simulink model "motor"  (R2017b)
settings: Solver=VariableStepAuto  StartTime=0.0  StopTime=12  FixedStep=0.001  RelTol=1e-3
undefined symbols (not defined in the file or in its folder): Amp1d, Amp1n, AmpSat1, BackEMF1, DiscIntNeverNeededParam, Elec1d, Elec1n, Mech1d, Mech1n, NomCurrent, PWMConversion, StallCurrent, StaticFric, TConst1
libraries: simulink x10
settings Model: SimulationMode=accelerator  Creator=Moochster  LastModifiedBy=lucyl

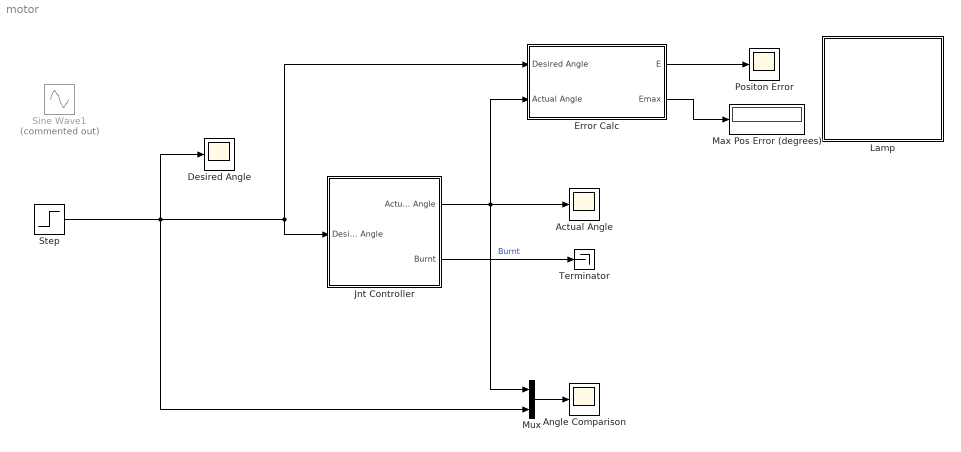
== system motor ==
  Actual Angle : Scope
  Angle Comparison : Scope
  Desired Angle : Scope
  Error Calc : Subsystem
  Jnt Controller : Subsystem
  Lamp : Subsystem  DialogController=hmiCreateDDGDialog  IsWebBlock=on  mask(MWDashboardBlock){webBlockId=7fcfd6b5-b98b-441a-9880-35fe4990fbef, webBlockType=lamp, ShowInLibBrowser=on, ShowInitialText=on, HMISrcModelName=motor}
      mask prompts: webBlockType "WebBlock Type"; HMISrcModelName "Source Model"
      mask help: SimulinkHMI:dialogs:LampDialogDesc
      mask Help: helpview([docroot '/mapfiles/simulink.map'], 'hmi_lamp')
      mask Display:
      | if strcmp(get_param(bdroot(gcb),'BlockDiagramType'), 'library')
      |     image([(matlabroot) '/toolbox/simulink/hmi/icons/Lamp.png']);
      | end
  Max Pos Error (degrees) : Display
  Mux : Mux  Inputs=2
  Positon Error : Scope
  Sine Wave1 : Sin  Commented=on  Amplitude=pi/4  Frequency=15*2*pi  Samples=15  SampleTime=0
  Step : Step  Time=0.02  SampleTime=0
  Terminator : Terminator
  wires:
  Step/1 -> Mux/2, Desired Angle/1, Error Calc/1(Desired Angle), Jnt Controller/1(Desired Angle)
  Jnt Controller/1(Actual Angle) -> Error Calc/2(Actual Angle), Actual Angle/1, Mux/1
  Error Calc/1(E) -> Positon Error/1
  Error Calc/2(Emax) -> Max Pos Error (degrees)/1
  Jnt Controller/2(Burnt) -> Terminator/1  "Burnt"
  Mux/1 -> Angle Comparison/1

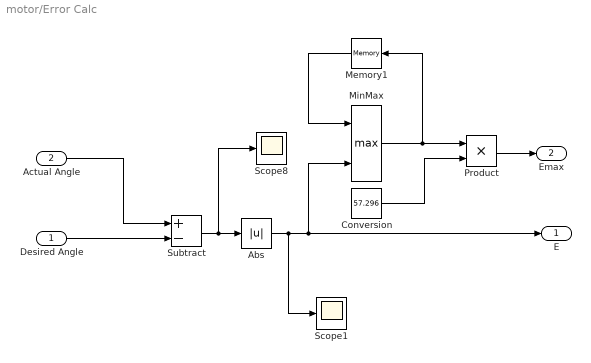
== system motor/Error Calc ==
  Desired Angle : Inport
  Actual Angle : Inport  Port=2
  Abs : Abs
  Conversion : Constant  Value=57.296
  Memory1 : Memory
  MinMax : MinMax  Function=max  Inputs=2  ZeroCross=off
  Product : Product
  Scope1 : Scope
  Scope8 : Scope
  Subtract : Sum  Inputs=+-
  E : Outport
  Emax : Outport  Port=2
  wires:
  Actual Angle/1 -> Subtract/1
  Desired Angle/1 -> Subtract/2
  Subtract/1 -> Scope8/1, Abs/1
  MinMax/1 -> Product/1, Memory1/1
  Memory1/1 -> MinMax/1
  Abs/1 -> Scope1/1, MinMax/2, E/1
  Product/1 -> Emax/1
  Conversion/1 -> Product/2

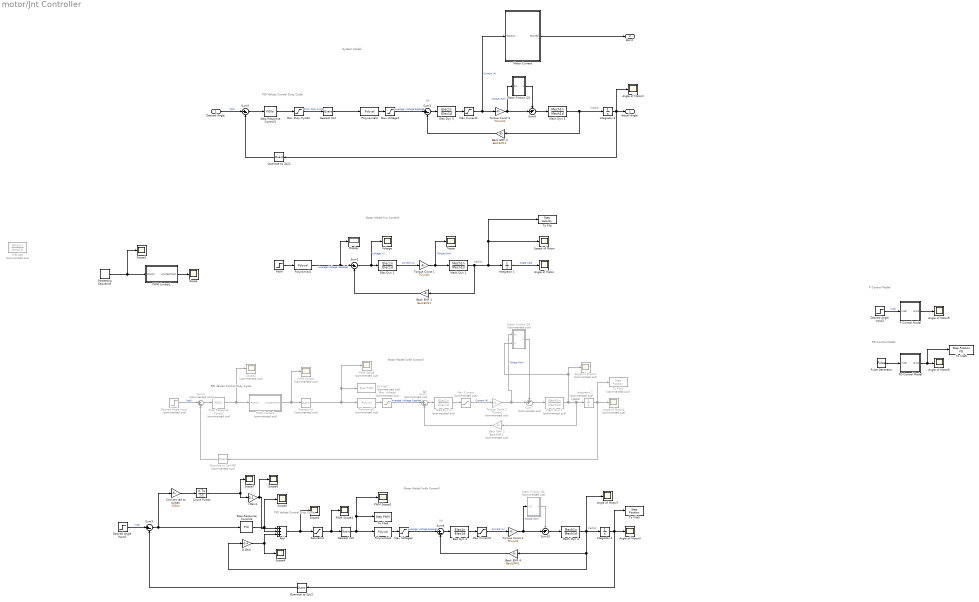
== system motor/Jnt Controller ==
  note: (rad/s)
  note: (rad/s)
  note: (V)
  note: PID Values Control Duty Cycle
  note: Motor Model (no Control)
  note: Motor Model (with Control)
  note: System Model
  note: (rad/s)
  note: (V)
  note: PID Values Control Duty Cycle
  note: (rad/s)
  note: (V)
  note: PID Values Control Duty Cycle
  note: Motor Model (with Control)
  note: P Control Model
  note: PD Control Model
  Desired Angle : Inport
  Add : Sum  Inputs=+++
  Angle of Motor{,2..3,5..7} (6 alike) : Scope
  Angle of Motor1 : Scope  Commented=on
  Angle of Motor4 : Scope  Commented=on
  Back EMF 1 : Gain  Gain=BackEMF1
  Back EMF 2 : Gain  Commented=on  Gain=BackEMF1
  Back EMF 3 : Gain  Gain=BackEMF1
  Back EMF 4 : Gain  Gain=BackEMF1
  Convert rad to pulses : Gain  Gain=200/pi
  Count Pulses : DiscreteIntegrator  InitialConditionSetting=State (most efficient)  SampleTime=0.001  ICPrevOutput=DiscIntNeverNeededParam  ICPrevScaledInput=DiscIntNeverNeededParam
  D Gain : Gain  Gain=-0.4
  Desired Angle Input : Step  Commented=on  Time=0  After=pi  SampleTime=0
  Desired Angle Input1 : Step  Time=0  After=pi  SampleTime=0
  Desired Angle Input2 : Step  Time=0  After=4*pi  SampleTime=0
  Display : Display
  Elec Dyn 1 : TransferFcn  Numerator=Elec1n  Denominator=Elec1d
  Elec Dyn 2 : TransferFcn  Commented=on  Numerator=Elec1n  Denominator=Elec1d
  Elec Dyn 3 : TransferFcn  Numerator=Elec1n  Denominator=Elec1d
  Elec Dyn 4 : TransferFcn  Numerator=Elec1n  Denominator=Elec1d
  "H-Bridge " : TransferFcn  Commented=on  Numerator=Amp1n  Denominator=Amp1d
  I Gain1 : Gain  Gain=0.1
  Integrator 1 : Integrator
  Integrator 2 : Integrator  Commented=on
  Integrator 3 : Integrator
  Integrator 4 : Integrator
  Max Current : Saturate  Commented=on  UpperLimit=1  LowerLimit=-1
  Max Current1 : Saturate  UpperLimit=1  LowerLimit=-1
  Max Current2 : Saturate  UpperLimit=1  LowerLimit=-1
  Max Duty Cycle2 : Saturate  UpperLimit=255  LowerLimit=-255
  Max Voltage : Saturate  Commented=on  UpperLimit=AmpSat1  LowerLimit=-AmpSat1
  Max Voltage1 : Saturate  UpperLimit=AmpSat1  LowerLimit=-AmpSat1
  Max Voltage2 : Saturate  UpperLimit=AmpSat1  LowerLimit=-AmpSat1
  Mech Dyn 1 : TransferFcn  Numerator=Mech1n  Denominator=Mech1d
  Mech Dyn 2 : TransferFcn  Commented=on  Numerator=Mech1n  Denominator=Mech1d
  Mech Dyn 3 : TransferFcn  Numerator=Mech1n  Denominator=Mech1d
  Mech Dyn 4 : TransferFcn  Numerator=Mech1n  Denominator=Mech1d
  Motor Current : Subsystem
  Nearest Int : Quantizer  Commented=on  QuantizationInterval=1
  Nearest Int1 : Quantizer  QuantizationInterval=1
  Nearest Int2 : Quantizer  QuantizationInterval=1
  "P Control Model " : Subsystem
  PD Control Model : Subsystem
  PWM : Step  Time=0.02  After=25  SampleTime=0
  PWM Limiter1 : Subsystem
  PWM Limiter2 : Subsystem  Commented=on
  PWM Scope : Scope  Commented=on
  PWM Scope1 : Scope  Commented=on
  PWM Scope2 : Scope
  PWM Scope3 : Scope
  Polynomial1 : Polyval  Coefs=PWMConversion
  Polynomial2 : Polyval  Commented=on  Coefs=PWMConversion
  Polynomial3 : Polyval  Coefs=PWMConversion
  Polynomial4 : Polyval  Coefs=PWMConversion
  Pulse Generator : DiscretePulseGenerator  PulseType=Time based  Amplitude=pi  Period=4  PulseWidth=50  PhaseDelay=0.5
  Quantize to 2pi/1 : Quantizer  QuantizationInterval=2*pi/400
  Quantize to 2pi/2 : Quantizer  QuantizationInterval=2*pi/400
  Quantize to 2pi/400 : Quantizer  Commented=on  QuantizationInterval=2*pi/400
  Repeating Sequence : simulink/Sources/Repeating Sequence  rep_seq_t=[0 2]  rep_seq_y=[-255 255]
  Saturation : Saturate  UpperLimit=255  LowerLimit=-255
  Scope{,1,3..7} (7 alike) : Scope
  Scope2 : Scope  Commented=on
  Speed of Motor : Scope
  Static Friction Q1 : Subsystem  Commented=on
  Static Friction Q2 : Subsystem
  Static Friction Q4 : Subsystem  Commented=on
  Step Response Control : simulink/Continuous/PID Controller  Commented=on  Controller=PID  TimeDomain=Continuous-time  SampleTime=-1  IntegratorMethod=Backward Euler  FilterMethod=Backward Euler  Form=Parallel  UseFilter=on  ControllerParametersSource=internal  P=10/pi  I=0  D=0  N=12783.9693192408  InitialConditionSource=internal  InitialConditionForIntegrator=0  InitialConditionForFilter=0  ExternalReset=none  LimitOutput=off  UpperSaturationLimit=inf  LowerSaturationLimit=-inf  LinearizeAsGain=on  AntiWindupMode=none  Kb=1  TrackingMode=off  Kt=1  PParamMin=[]  PParamMax=[]  IParamMin=[]  IParamMax=[]  DParamMin=[]  DParamMax=[]  NParamMin=[]  NParamMax=[]  KbParamMin=[]  KbParamMax=[]  KtParamMin=[]  KtParamMax=[]  POutMin=[]  POutMax=[]  IOutMin=[]  IOutMax=[]  DOutMin=[]  DOutMax=[]  NOutMin=[]  NOutMax=[]  KbOutMin=[]  KbOutMax=[]  KtOutMin=[]  KtOutMax=[]  IntegratorOutMin=[]  IntegratorOutMax=[]  FilterOutMin=[]  FilterOutMax=[]  SumOutMin=[]  SumOutMax=[]  SumI1OutMin=[]  SumI1OutMax=[]  SumI2OutMin=[]  SumI2OutMax=[]  SumI3OutMin=[]  SumI3OutMax=[]  SumDOutMin=[]  SumDOutMax=[]  SaturationOutMin=[]  SaturationOutMax=[]  IntegratorContinuousStateAttributes=''  IntegratorStateMustResolveToSignalObject=off  IntegratorRTWStateStorageClass=Auto  FilterContinuousStateAttributes=''  FilterStateMustResolveToSignalObject=off  FilterRTWStateStorageClass=Auto  DifferentiatorICPrevScaledInput=0  DifferentiatorOutMin=[]  DifferentiatorOutMax=[]  InitialConditionSetting=State (most efficient)  FilterDiffOutCoefMin=[]  FilterDiffOutCoefMax=[]  SumDenOutMin=[]  SumDenOutMax=[]  SumNumOutMin=[]  SumNumOutMax=[]  ReciprocalOutMin=[]  ReciprocalOutMax=[]  DivideOutMin=[]  DivideOutMax=[]  TunerSelectOption=Transfer Function Based (PID Tuner App)
  Step Response Control1 : simulink/Continuous/PID Controller  Controller=PID  TimeDomain=Continuous-time  SampleTime=-1  IntegratorMethod=Forward Euler  FilterMethod=Forward Euler  Form=Parallel  UseFilter=on  ControllerParametersSource=internal  P=10/pi  I=0  D=0  N=12783.9693192408  InitialConditionSource=internal  InitialConditionForIntegrator=0  InitialConditionForFilter=0  ExternalReset=none  LimitOutput=off  UpperSaturationLimit=inf  LowerSaturationLimit=-inf  LinearizeAsGain=on  AntiWindupMode=none  Kb=1  TrackingMode=off  Kt=1  PParamMin=[]  PParamMax=[]  IParamMin=[]  IParamMax=[]  DParamMin=[]  DParamMax=[]  NParamMin=[]  NParamMax=[]  KbParamMin=[]  KbParamMax=[]  KtParamMin=[]  KtParamMax=[]  POutMin=[]  POutMax=[]  IOutMin=[]  IOutMax=[]  DOutMin=[]  DOutMax=[]  NOutMin=[]  NOutMax=[]  KbOutMin=[]  KbOutMax=[]  KtOutMin=[]  KtOutMax=[]  IntegratorOutMin=[]  IntegratorOutMax=[]  FilterOutMin=[]  FilterOutMax=[]  SumOutMin=[]  SumOutMax=[]  SumI1OutMin=[]  SumI1OutMax=[]  SumI2OutMin=[]  SumI2OutMax=[]  SumI3OutMin=[]  SumI3OutMax=[]  SumDOutMin=[]  SumDOutMax=[]  SaturationOutMin=[]  SaturationOutMax=[]  IntegratorContinuousStateAttributes=''  IntegratorStateMustResolveToSignalObject=off  IntegratorRTWStateStorageClass=Auto  FilterContinuousStateAttributes=''  FilterStateMustResolveToSignalObject=off  FilterRTWStateStorageClass=Auto  DifferentiatorICPrevScaledInput=0  DifferentiatorOutMin=[]  DifferentiatorOutMax=[]  InitialConditionSetting=State (most efficient)  FilterDiffOutCoefMin=[]  FilterDiffOutCoefMax=[]  SumDenOutMin=[]  SumDenOutMax=[]  SumNumOutMin=[]  SumNumOutMax=[]  ReciprocalOutMin=[]  ReciprocalOutMax=[]  DivideOutMin=[]  DivideOutMax=[]  TunerSelectOption=Transfer Function Based (PID Tuner App)
  Step Response Control3 : simulink/Continuous/PID Controller  Controller=P  TimeDomain=Continuous-time  SampleTime=-1  IntegratorMethod=Backward Euler  FilterMethod=Backward Euler  Form=Parallel  UseFilter=on  ControllerParametersSource=internal  P=17.2248010753834  I=30.2607202690595  D=2.6356  N=6709.12247034215  InitialConditionSource=internal  InitialConditionForIntegrator=0  InitialConditionForFilter=0  ExternalReset=none  LimitOutput=off  UpperSaturationLimit=inf  LowerSaturationLimit=-inf  LinearizeAsGain=on  AntiWindupMode=none  Kb=1  TrackingMode=off  Kt=1  PParamMin=[]  PParamMax=[]  IParamMin=[]  IParamMax=[]  DParamMin=[]  DParamMax=[]  NParamMin=[]  NParamMax=[]  KbParamMin=[]  KbParamMax=[]  KtParamMin=[]  KtParamMax=[]  POutMin=[]  POutMax=[]  IOutMin=[]  IOutMax=[]  DOutMin=[]  DOutMax=[]  NOutMin=[]  NOutMax=[]  KbOutMin=[]  KbOutMax=[]  KtOutMin=[]  KtOutMax=[]  IntegratorOutMin=[]  IntegratorOutMax=[]  FilterOutMin=[]  FilterOutMax=[]  SumOutMin=[]  SumOutMax=[]  SumI1OutMin=[]  SumI1OutMax=[]  SumI2OutMin=[]  SumI2OutMax=[]  SumI3OutMin=[]  SumI3OutMax=[]  SumDOutMin=[]  SumDOutMax=[]  SaturationOutMin=[]  SaturationOutMax=[]  IntegratorContinuousStateAttributes=''  IntegratorStateMustResolveToSignalObject=off  IntegratorRTWStateStorageClass=Auto  FilterContinuousStateAttributes=''  FilterStateMustResolveToSignalObject=off  FilterRTWStateStorageClass=Auto  DifferentiatorICPrevScaledInput=0  DifferentiatorOutMin=[]  DifferentiatorOutMax=[]  InitialConditionSetting=State (most efficient)  FilterDiffOutCoefMin=[]  FilterDiffOutCoefMax=[]  SumDenOutMin=[]  SumDenOutMax=[]  SumNumOutMin=[]  SumNumOutMax=[]  ReciprocalOutMin=[]  ReciprocalOutMax=[]  DivideOutMin=[]  DivideOutMax=[]  TunerSelectOption=Transfer Function Based (PID Tuner App)
  Sum{1,3,5,8..9} (5 alike) : Sum  Inputs=|+-
  Sum10 : Sum  Inputs=-+|
  Sum2 : Sum  Commented=on  Inputs=|+-
  Sum4 : Sum  Commented=on  Inputs=|+-
  Sum6 : Sum  Inputs=-+|
  Sum7 : Sum  Commented=on  Inputs=-+|
  Tester : Scope
  To File : ToFile  Filename=Step Velocity  SampleTime=0.01
  To File1 : ToFile  Commented=on  Filename=Step Position  SampleTime=0.01
  To File2 : ToFile  Commented=on  Filename=Step PWM  SampleTime=0.01
  To File3 : ToFile  Filename=Step Position  SampleTime=0.01
  To File4 : ToFile  Filename=Step PWM  SampleTime=0.01
  To File5 : ToFile  Filename=Step Position PD  SampleTime=0.01
  Torque Const 1 : Gain  Gain=TConst1
  Torque Const 2 : Gain  Commented=on  Gain=TConst1
  Torque Const 3 : Gain  Gain=TConst1
  Torque Const 4 : Gain  Gain=TConst1
  Voltage : Scope
  Actual Angle : Outport
  Burnt : Outport  Port=2
  wires:
  Motor Current/1(Burned) -> Burnt/1
  Mech Dyn 1/1 -> Back EMF 1/1, Integrator 1/1, To File/1, Speed of Motor/1
  Integrator 1/1 -> Angle of Motor/1  "Angle (rad)"
  Torque Const 1/1 -> Tester/1, Mech Dyn 1/1  "Torque (Nm)"
  Back EMF 1/1 -> Sum1/2
  Elec Dyn 1/1 -> Torque Const 1/1  "Current (A)"
  Sum1/1 -> Elec Dyn 1/1, Voltage/1  "Voltage (V)"
  Max Voltage/1 -> Sum2/1  "Average  Voltage Supplied"
  Desired Angle Input/1 -> Sum4/1  "(rad)"
  Back EMF 2/1 -> Sum2/2
  Elec Dyn 2/1 -> Max Current/1
  Sum4/1 -> Step Response Control/1
  Sum2/1 -> Elec Dyn 2/1
  Step Response Control/1 -> PWM Limiter2/1(PWMIn), Scope2/1
  Polynomial1/1 -> Display/1, Sum1/1  "Average Voltage  Supplied"
  PWM/1 -> Polynomial1/1
  Polynomial2/1 -> Max Voltage/1
  Max Current/1 -> Torque Const 2/1  "Current (A)"
  Quantize to 2pi/400/1 -> Sum4/2
  Sum7/1 -> Mech Dyn 2/1
  Mech Dyn 2/1 -> Static Friction Q4/2(w), Angle of Motor4/1, Back EMF 2/1, Integrator 2/1
  Torque Const 2/1 -> Static Friction Q4/1(Fin), Sum7/2  "Torque (Nm)"
  Integrator 2/1 -> To File1/1, Angle of Motor1/1, Quantize to 2pi/400/1
  Static Friction Q2/1(Fout) -> Sum6/1
  Integrator 3/1 -> Actual Angle/1, Angle of Motor2/1, Quantize to 2pi/1/1
  Nearest Int1/1 -> Polynomial3/1
  Torque Const 3/1 -> Sum6/2, Static Friction Q2/1(Fin)  "Torque (Nm)"
  Mech Dyn 3/1 -> Integrator 3/1, Back EMF 3/1
  Sum6/1 -> Mech Dyn 3/1
  Quantize to 2pi/1/1 -> Sum5/2
  Max Current1/1 -> Motor Current/1(MotCurr), Torque Const 3/1  "Current (A)"
  Polynomial3/1 -> Max Voltage1/1
  Step Response Control1/1 -> Max Duty Cycle2/1
  Sum3/1 -> Elec Dyn 3/1
  Sum5/1 -> Step Response Control1/1
  Elec Dyn 3/1 -> Max Current1/1
  Back EMF 3/1 -> Sum3/2
  Desired Angle/1 -> Sum5/1  "(rad)"
  Max Voltage1/1 -> Sum3/1  "Average  Voltage Supplied"
  Max Duty Cycle2/1 -> Nearest Int1/1  "PWM  Duty Cycle"
  Repeating Sequence/1 -> PWM Limiter1/1(PWMIn), Scope1/1
  PWM Limiter1/1("Limited PWM ") -> Scope/1
  Nearest Int/1 -> PWM Scope/1, To File2/1, Polynomial2/1
  PWM Limiter2/1("Limited PWM ") -> PWM Scope1/1, Nearest Int/1
  Saturation/1 -> Nearest Int2/1, PWM Scope3/1
  Nearest Int2/1 -> Polynomial4/1, To File4/1, PWM Scope2/1
  Integrator 4/1 -> Quantize to 2pi/2/1, Angle of Motor3/1, To File3/1
  Torque Const 4/1 -> Static Friction Q1/1(Fin), Sum10/2  "Torque (Nm)"
  Mech Dyn 4/1 -> Angle of Motor7/1, D Gain/1, Back EMF 4/1, Integrator 4/1
  Sum10/1 -> Mech Dyn 4/1
  Quantize to 2pi/2/1 -> Sum9/2
  Max Current2/1 -> Torque Const 4/1  "Current (A)"
  Polynomial4/1 -> Max Voltage2/1
  Add/1 -> Saturation/1, Scope3/1
  Sum8/1 -> Elec Dyn 4/1
  Elec Dyn 4/1 -> Max Current2/1
  Back EMF 4/1 -> Sum8/2
  Desired Angle Input1/1 -> Sum9/1  "(rad)"
  Max Voltage2/1 -> Sum8/1  "Average  Voltage Supplied"
  Static Friction Q4/1(Fout) -> Sum7/1
  Static Friction Q1/1(Fout) -> Sum10/1
  Desired Angle Input2/1 -> "P Control Model "/1((rad))  "(rad)"
  "P Control Model "/1(Out1) -> Angle of Motor5/1
  Step Response Control3/1 -> Add/2, Scope5/1
  Sum9/1 -> Convert rad to pulses/1, Step Response Control3/1
  D Gain/1 -> Add/3, Scope4/1
  PD Control Model/1(Out1) -> To File5/1, Angle of Motor6/1
  Count Pulses/1 -> I Gain1/1, Scope7/1
  I Gain1/1 -> Scope6/1, Add/1
  Convert rad to pulses/1 -> Count Pulses/1
  Pulse Generator/1 -> PD Control Model/1((rad))

== system motor/Lamp ==

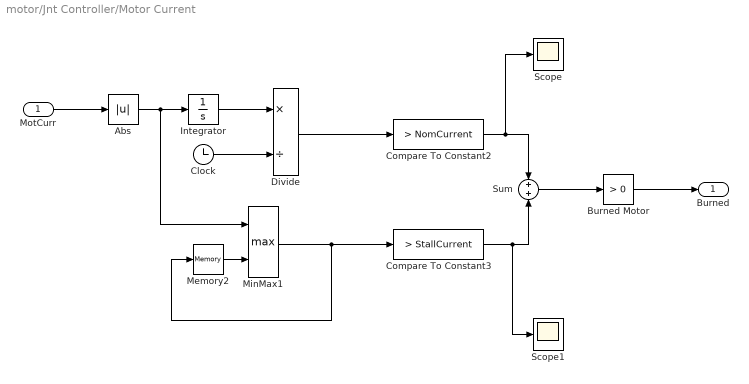
== system motor/Jnt Controller/Motor Current ==
  MotCurr : Inport
  Abs : Abs
  Burned Motor : simulink/Logic and Bit Operations/Compare To Zero  relop=>  OutDataTypeStr=boolean
  Clock : Clock
  Compare To Constant2 : simulink/Logic and Bit Operations/Compare To Constant  relop=>  const=NomCurrent  OutDataTypeStr=boolean
  Compare To Constant3 : simulink/Logic and Bit Operations/Compare To Constant  relop=>  const=StallCurrent  OutDataTypeStr=boolean
  Divide : Product  Inputs=*/
  Integrator : Integrator
  Memory2 : Memory
  MinMax1 : MinMax  Function=max  Inputs=2  ZeroCross=off
  Scope : Scope
  Scope1 : Scope
  Sum : Sum
  Burned : Outport
  wires:
  Sum/1 -> Burned Motor/1
  Burned Motor/1 -> Burned/1
  Memory2/1 -> MinMax1/2
  Compare To Constant2/1 -> Scope/1, Sum/1
  Compare To Constant3/1 -> Scope1/1, Sum/2
  MinMax1/1 -> Memory2/1, Compare To Constant3/1
  Divide/1 -> Compare To Constant2/1
  Abs/1 -> Integrator/1, MinMax1/1
  Clock/1 -> Divide/2
  Integrator/1 -> Divide/1
  MotCurr/1 -> Abs/1

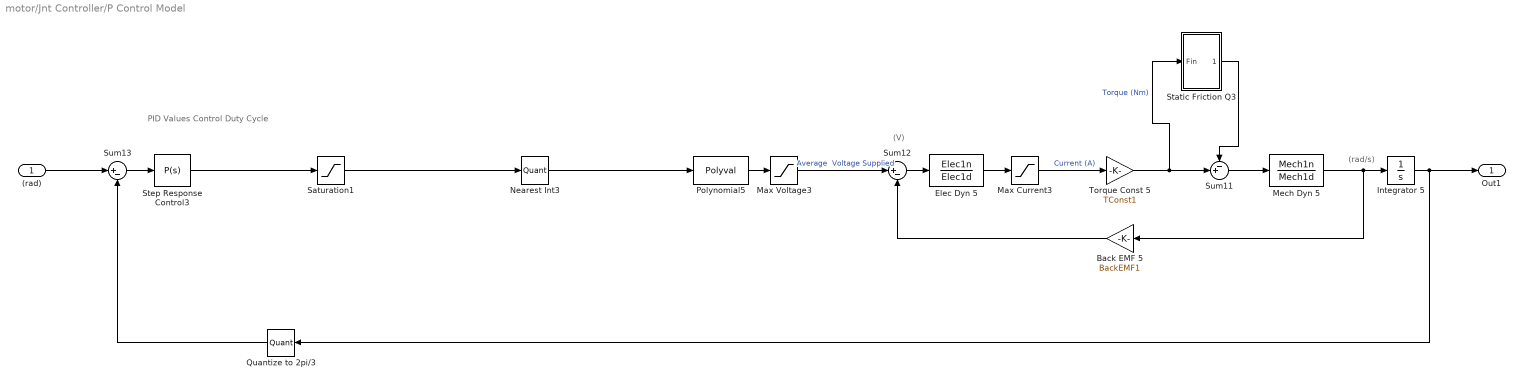
== system motor/Jnt Controller/P Control Model  ==
  note: (rad/s)
  note: (V)
  note: PID Values Control Duty Cycle
  (rad) : Inport
  Back EMF 5 : Gain  Gain=BackEMF1
  Elec Dyn 5 : TransferFcn  Numerator=Elec1n  Denominator=Elec1d
  Integrator 5 : Integrator
  Max Current3 : Saturate  UpperLimit=1  LowerLimit=-1
  Max Voltage3 : Saturate  UpperLimit=AmpSat1  LowerLimit=-AmpSat1
  Mech Dyn 5 : TransferFcn  Numerator=Mech1n  Denominator=Mech1d
  Nearest Int3 : Quantizer  QuantizationInterval=1
  Polynomial5 : Polyval  Coefs=PWMConversion
  Quantize to 2pi/3 : Quantizer  QuantizationInterval=2*pi/400
  Saturation1 : Saturate  UpperLimit=255  LowerLimit=-255
  Static Friction Q3 : Subsystem
  Step Response Control3 : simulink/Continuous/PID Controller  Controller=P  TimeDomain=Continuous-time  SampleTime=-1  IntegratorMethod=Backward Euler  FilterMethod=Backward Euler  Form=Parallel  UseFilter=on  ControllerParametersSource=internal  P=10/pi  I=65.9706798485148  D=4.84769528476857  N=6709.12247034215  InitialConditionSource=internal  InitialConditionForIntegrator=0  InitialConditionForFilter=0  ExternalReset=none  LimitOutput=off  UpperSaturationLimit=inf  LowerSaturationLimit=-inf  LinearizeAsGain=on  AntiWindupMode=none  Kb=1  TrackingMode=off  Kt=1  PParamMin=[]  PParamMax=[]  IParamMin=[]  IParamMax=[]  DParamMin=[]  DParamMax=[]  NParamMin=[]  NParamMax=[]  KbParamMin=[]  KbParamMax=[]  KtParamMin=[]  KtParamMax=[]  POutMin=[]  POutMax=[]  IOutMin=[]  IOutMax=[]  DOutMin=[]  DOutMax=[]  NOutMin=[]  NOutMax=[]  KbOutMin=[]  KbOutMax=[]  KtOutMin=[]  KtOutMax=[]  IntegratorOutMin=[]  IntegratorOutMax=[]  FilterOutMin=[]  FilterOutMax=[]  SumOutMin=[]  SumOutMax=[]  SumI1OutMin=[]  SumI1OutMax=[]  SumI2OutMin=[]  SumI2OutMax=[]  SumI3OutMin=[]  SumI3OutMax=[]  SumDOutMin=[]  SumDOutMax=[]  SaturationOutMin=[]  SaturationOutMax=[]  IntegratorContinuousStateAttributes=''  IntegratorStateMustResolveToSignalObject=off  IntegratorRTWStateStorageClass=Auto  FilterContinuousStateAttributes=''  FilterStateMustResolveToSignalObject=off  FilterRTWStateStorageClass=Auto  DifferentiatorICPrevScaledInput=0  DifferentiatorOutMin=[]  DifferentiatorOutMax=[]  InitialConditionSetting=State (most efficient)  FilterDiffOutCoefMin=[]  FilterDiffOutCoefMax=[]  SumDenOutMin=[]  SumDenOutMax=[]  SumNumOutMin=[]  SumNumOutMax=[]  ReciprocalOutMin=[]  ReciprocalOutMax=[]  DivideOutMin=[]  DivideOutMax=[]  TunerSelectOption=Transfer Function Based (PID Tuner App)
  Sum11 : Sum  Inputs=-+|
  Sum12 : Sum  Inputs=|+-
  Sum13 : Sum  Inputs=|+-
  Torque Const 5 : Gain  Gain=TConst1
  Out1 : Outport
  wires:
  Sum11/1 -> Mech Dyn 5/1
  Mech Dyn 5/1 -> Integrator 5/1, Back EMF 5/1
  Integrator 5/1 -> Out1/1, Quantize to 2pi/3/1
  Nearest Int3/1 -> Polynomial5/1
  Saturation1/1 -> Nearest Int3/1
  Quantize to 2pi/3/1 -> Sum13/2
  Sum13/1 -> Step Response Control3/1
  Torque Const 5/1 -> Sum11/2, Static Friction Q3/1(Fin)  "Torque (Nm)"
  Static Friction Q3/1(Fout) -> Sum11/1
  Elec Dyn 5/1 -> Max Current3/1
  Max Current3/1 -> Torque Const 5/1  "Current (A)"
  (rad)/1 -> Sum13/1
  Back EMF 5/1 -> Sum12/2
  Sum12/1 -> Elec Dyn 5/1
  Step Response Control3/1 -> Saturation1/1
  Max Voltage3/1 -> Sum12/1  "Average  Voltage Supplied"
  Polynomial5/1 -> Max Voltage3/1

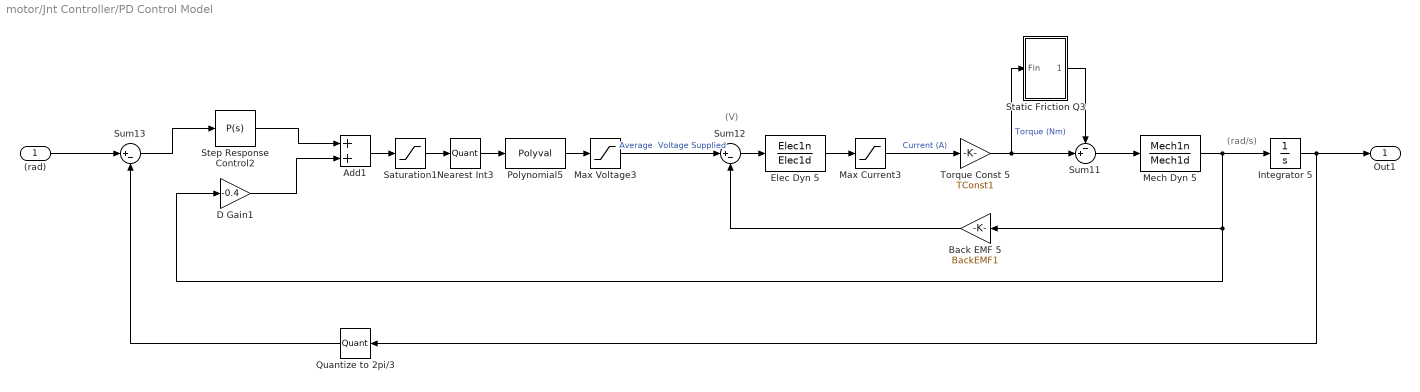
== system motor/Jnt Controller/PD Control Model ==
  note: (rad/s)
  note: (V)
  (rad) : Inport
  Add1 : Sum
  Back EMF 5 : Gain  Gain=BackEMF1
  D Gain1 : Gain  Gain=-0.4
  Elec Dyn 5 : TransferFcn  Numerator=Elec1n  Denominator=Elec1d
  Integrator 5 : Integrator
  Max Current3 : Saturate  UpperLimit=1  LowerLimit=-1
  Max Voltage3 : Saturate  UpperLimit=AmpSat1  LowerLimit=-AmpSat1
  Mech Dyn 5 : TransferFcn  Numerator=Mech1n  Denominator=Mech1d
  Nearest Int3 : Quantizer  QuantizationInterval=1
  Polynomial5 : Polyval  Coefs=PWMConversion
  Quantize to 2pi/3 : Quantizer  QuantizationInterval=2*pi/400
  Saturation1 : Saturate  UpperLimit=255  LowerLimit=-255
  Static Friction Q3 : Subsystem
  Step Response Control2 : simulink/Continuous/PID Controller  Controller=P  TimeDomain=Continuous-time  SampleTime=-1  IntegratorMethod=Backward Euler  FilterMethod=Backward Euler  Form=Parallel  UseFilter=on  ControllerParametersSource=internal  P=17.7  I=65.9706798485148  D=2.6356  N=6709.12247034215  InitialConditionSource=internal  InitialConditionForIntegrator=0  InitialConditionForFilter=0  ExternalReset=none  LimitOutput=off  UpperSaturationLimit=inf  LowerSaturationLimit=-inf  LinearizeAsGain=on  AntiWindupMode=none  Kb=1  TrackingMode=off  Kt=1  PParamMin=[]  PParamMax=[]  IParamMin=[]  IParamMax=[]  DParamMin=[]  DParamMax=[]  NParamMin=[]  NParamMax=[]  KbParamMin=[]  KbParamMax=[]  KtParamMin=[]  KtParamMax=[]  POutMin=[]  POutMax=[]  IOutMin=[]  IOutMax=[]  DOutMin=[]  DOutMax=[]  NOutMin=[]  NOutMax=[]  KbOutMin=[]  KbOutMax=[]  KtOutMin=[]  KtOutMax=[]  IntegratorOutMin=[]  IntegratorOutMax=[]  FilterOutMin=[]  FilterOutMax=[]  SumOutMin=[]  SumOutMax=[]  SumI1OutMin=[]  SumI1OutMax=[]  SumI2OutMin=[]  SumI2OutMax=[]  SumI3OutMin=[]  SumI3OutMax=[]  SumDOutMin=[]  SumDOutMax=[]  SaturationOutMin=[]  SaturationOutMax=[]  IntegratorContinuousStateAttributes=''  IntegratorStateMustResolveToSignalObject=off  IntegratorRTWStateStorageClass=Auto  FilterContinuousStateAttributes=''  FilterStateMustResolveToSignalObject=off  FilterRTWStateStorageClass=Auto  DifferentiatorICPrevScaledInput=0  DifferentiatorOutMin=[]  DifferentiatorOutMax=[]  InitialConditionSetting=State (most efficient)  FilterDiffOutCoefMin=[]  FilterDiffOutCoefMax=[]  SumDenOutMin=[]  SumDenOutMax=[]  SumNumOutMin=[]  SumNumOutMax=[]  ReciprocalOutMin=[]  ReciprocalOutMax=[]  DivideOutMin=[]  DivideOutMax=[]  TunerSelectOption=Transfer Function Based (PID Tuner App)
  Sum11 : Sum  Inputs=-+|
  Sum12 : Sum  Inputs=|+-
  Sum13 : Sum  Inputs=|+-
  Torque Const 5 : Gain  Gain=TConst1
  Out1 : Outport
  wires:
  Sum13/1 -> Step Response Control2/1
  Step Response Control2/1 -> Add1/1
  Static Friction Q3/1(Fout) -> Sum11/1
  Back EMF 5/1 -> Sum12/2
  (rad)/1 -> Sum13/1
  Add1/1 -> Saturation1/1
  Polynomial5/1 -> Max Voltage3/1
  Sum12/1 -> Elec Dyn 5/1
  Max Current3/1 -> Torque Const 5/1  "Current (A)"
  Max Voltage3/1 -> Sum12/1  "Average  Voltage Supplied"
  D Gain1/1 -> Add1/2
  Sum11/1 -> Mech Dyn 5/1
  Quantize to 2pi/3/1 -> Sum13/2
  Mech Dyn 5/1 -> Integrator 5/1, Back EMF 5/1, D Gain1/1
  Integrator 5/1 -> Out1/1, Quantize to 2pi/3/1
  Elec Dyn 5/1 -> Max Current3/1
  Torque Const 5/1 -> Sum11/2, Static Friction Q3/1(Fin)  "Torque (Nm)"
  Nearest Int3/1 -> Polynomial5/1
  Saturation1/1 -> Nearest Int3/1

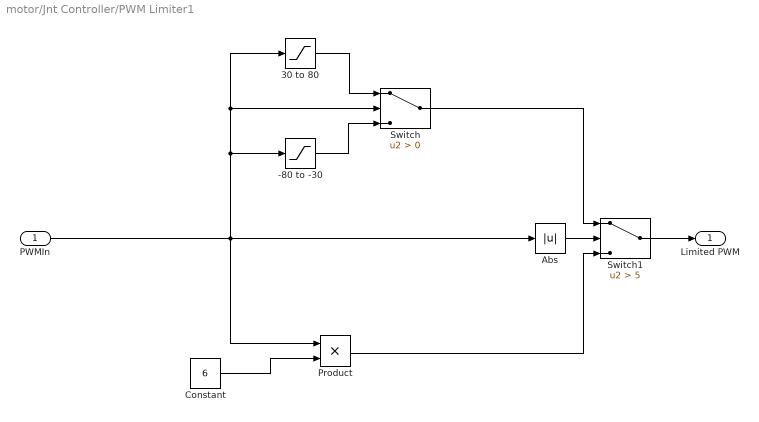
== system motor/Jnt Controller/PWM Limiter1 ==
  PWMIn : Inport
  -80 to -30 : Saturate  UpperLimit=-30  LowerLimit=-80  RndMeth=Nearest
  30 to 80 : Saturate  UpperLimit=80  LowerLimit=30  RndMeth=Round
  Abs : Abs
  Constant : Constant  Value=6
  Product : Product
  Switch : Switch  Criteria=u2 > Threshold
  Switch1 : Switch  Criteria=u2 > Threshold  Threshold=5
  "Limited PWM " : Outport
  wires:
  Switch1/1 -> "Limited PWM "/1
  Product/1 -> Switch1/3
  Constant/1 -> Product/2
  Switch/1 -> Switch1/1
  Abs/1 -> Switch1/2
  PWMIn/1 -> -80 to -30/1, Switch/2, 30 to 80/1, Abs/1, Product/1
  -80 to -30/1 -> Switch/3
  30 to 80/1 -> Switch/1

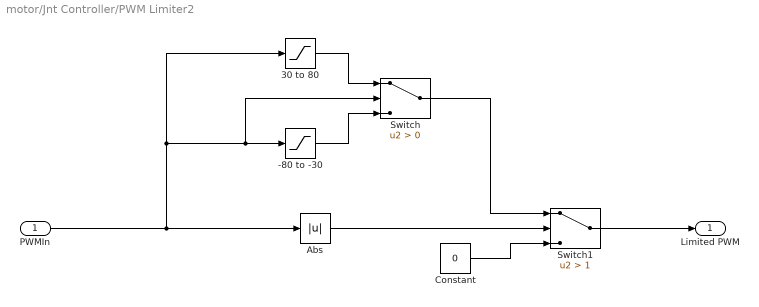
== system motor/Jnt Controller/PWM Limiter2 ==
  PWMIn : Inport
  -80 to -30 : Saturate  UpperLimit=-25  LowerLimit=-80  RndMeth=Nearest
  30 to 80 : Saturate  UpperLimit=80  LowerLimit=25  RndMeth=Round
  Abs : Abs
  Constant : Constant  Value=0
  Switch : Switch  Criteria=u2 > Threshold
  Switch1 : Switch  Criteria=u2 > Threshold  Threshold=1
  "Limited PWM " : Outport
  wires:
  30 to 80/1 -> Switch/1
  -80 to -30/1 -> Switch/3
  PWMIn/1 -> 30 to 80/1, Switch/2, -80 to -30/1, Abs/1
  Abs/1 -> Switch1/2
  Constant/1 -> Switch1/3
  Switch/1 -> Switch1/1
  Switch1/1 -> "Limited PWM "/1

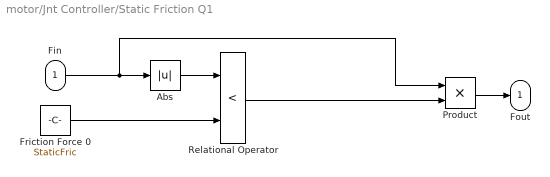
== system motor/Jnt Controller/Static Friction Q1 ==
  Fin : Inport
  Abs : Abs  ZeroCross=off
  Friction Force 0 : Constant  Value=StaticFric
  Product : Product
  Relational Operator : RelationalOperator  Operator=<  OutDataTypeStr=boolean  ZeroCross=off  RndMeth=Simplest
  Fout : Outport
  wires:
  Abs/1 -> Relational Operator/1
  Fin/1 -> Product/1, Abs/1
  Product/1 -> Fout/1
  Friction Force 0/1 -> Relational Operator/2
  Relational Operator/1 -> Product/2

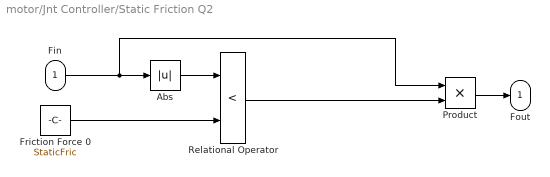
== system motor/Jnt Controller/Static Friction Q2 ==
  Fin : Inport
  Abs : Abs
  Friction Force 0 : Constant  Value=StaticFric
  Product : Product
  Relational Operator : RelationalOperator  Operator=<  OutDataTypeStr=boolean  RndMeth=Simplest
  Fout : Outport
  wires:
  Relational Operator/1 -> Product/2
  Friction Force 0/1 -> Relational Operator/2
  Product/1 -> Fout/1
  Fin/1 -> Abs/1, Product/1
  Abs/1 -> Relational Operator/1

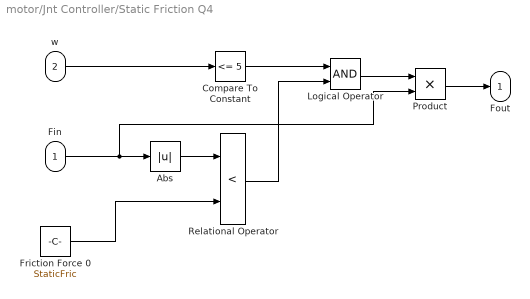
== system motor/Jnt Controller/Static Friction Q4 ==
  Fin : Inport
  w : Inport  Port=2
  Abs : Abs
  Compare To Constant : simulink/Logic and Bit Operations/Compare To Constant  relop=<=  const=5  OutDataTypeStr=boolean
  Friction Force 0 : Constant  Value=StaticFric
  Logical Operator : Logic  AllPortsSameDT=off  OutDataTypeStr=boolean
  Product : Product
  Relational Operator : RelationalOperator  Operator=<  OutDataTypeStr=boolean  ZeroCross=off  RndMeth=Simplest
  Fout : Outport
  wires:
  Friction Force 0/1 -> Relational Operator/2
  Product/1 -> Fout/1
  Compare To Constant/1 -> Logical Operator/1
  Relational Operator/1 -> Logical Operator/2
  Logical Operator/1 -> Product/1
  Fin/1 -> Product/2, Abs/1
  w/1 -> Compare To Constant/1
  Abs/1 -> Relational Operator/1

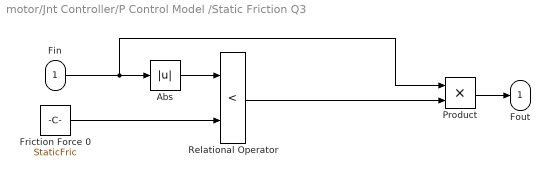
== system motor/Jnt Controller/P Control Model /Static Friction Q3 ==
  Fin : Inport
  Abs : Abs  ZeroCross=off
  Friction Force 0 : Constant  Value=StaticFric
  Product : Product
  Relational Operator : RelationalOperator  Operator=<  OutDataTypeStr=boolean  ZeroCross=off  RndMeth=Simplest
  Fout : Outport
  wires:
  Relational Operator/1 -> Product/2
  Friction Force 0/1 -> Relational Operator/2
  Product/1 -> Fout/1
  Fin/1 -> Abs/1, Product/1
  Abs/1 -> Relational Operator/1

== system motor/Jnt Controller/PD Control Model/Static Friction Q3 ==
  Fin : Inport
  Abs : Abs  ZeroCross=off
  Friction Force 0 : Constant  Value=StaticFric
  Product : Product
  Relational Operator : RelationalOperator  Operator=<  OutDataTypeStr=boolean  ZeroCross=off  RndMeth=Simplest
  Fout : Outport
  wires:
  Relational Operator/1 -> Product/2
  Friction Force 0/1 -> Relational Operator/2
  Product/1 -> Fout/1
  Fin/1 -> Abs/1, Product/1
  Abs/1 -> Relational Operator/1
